simulink model "ZSM_TeslaModelS_statKreisfahrt"  (R2020b)
settings: Solver=FixedStepDiscrete  StartTime=0.0  StopTime=simtime  FixedStep=stepsize  RelTol=1e-3
undefined symbols (not defined in the file): activate_stop, activate_stop_vmax, ay_stop, ayObs, ayStiff, Bat_param, deltav_ist, DiscIntNeverNeededParam, EG_wunsch, magnitude, mu_road_LF, mu_road_LR, mu_road_RF, mu_road_RR, par_ASR, par_MDT, par_TIR, par_VEH, select_delta_h, select_M_wheel, stepsize, t, temp_betriebsstrategie, temperature_LTrange, track_left, track_right
libraries: Library_ASK x36, simulink x16, pid_lib x2, dspstat3 x2, Library_Betriebsstrategie x2, vehicle_model x2, pacejka_trans x1
(part 1 of 7)
settings Model: SimulationMode=accelerator  ExtModeTrigDuration=100  TunableVars=activate_stop,ay_stop,par_TIR,par_VEH,select_M_wheel_final,select_M_wheel_initial,select_M_wheel_time,select_delta_h_final,select_delta_h_initial,select_delta_h_time,v0  TunableVarsStorageClass=Auto,Auto,Auto,Auto,Auto,Auto,Auto,Auto,Auto,Auto,Auto  TunableVarsTypeQualifier=,,,,,,,,,,  Creator=schultze  LastModifiedBy=ga69qig
settings DataIOCC: ExternalInput=input_data  LoadExternalInput=on  SaveFormat=StructureWithTime  SaveOutput=off  DSMLogging=off  SaveTime=off  ReturnWorkspaceOutputs=off  StateSaveName=tmp_raccel_xout  SignalLoggingName=tmp_raccel_logsout
settings OptimizationCC: DefaultParameterBehavior=Inlined  ExpressionDepthLimit=2147483647  EfficientMapNaN2IntZero=off  LifeSpan=inf  SimCompilerOptimization=on
settings DebuggingCC: SignalInfNanChecking=warning  ReadBeforeWriteMsg=DisableAll  WriteAfterWriteMsg=DisableAll  WriteAfterReadMsg=DisableAll  AlgebraicLoopMsg=none  ArtificialAlgebraicLoopMsg=none  UnderspecifiedInitializationDetection=Classic  SolverPrmCheckMsg=warning  MultiTaskDSMMsg=warning  MultiTaskCondExecSysMsg=none  FcnCallInpInsideContextMsg=warning  UnconnectedInputMsg=none  UnconnectedOutputMsg=none  UnconnectedLineMsg=none  AllowSymbolicDim=off  StateNameClashWarn=warning  NonBusSignalsTreatedAsBus=warning  SFUnexpectedBacktrackingDiag=warning  SFNoUnconditionalDefaultTransitionDiag=warning  SFExecutionAtInitializationDiag=none  ArithmeticOperatorsInVariantConditions=warning
settings HardwareCC: ProdBitPerPointer=32  ProdBitPerSizeT=32  ProdBitPerPtrDiffT=32  ProdLargestAtomicFloat=None  ProdIntDivRoundTo=Undefined  ProdEndianess=Unspecified  ProdWordSize=32  ProdHWDeviceType=Generic->Unspecified (assume 32-bit Generic)  TargetBitPerPointer=64  TargetBitPerSizeT=64  TargetBitPerPtrDiffT=64  TargetLongLongMode=on  TargetIntDivRoundTo=Zero  TargetEndianess=LittleEndian  TargetWordSize=64  TargetHWDeviceType=MATLAB Host  ProdEqTarget=off
settings ModelReferenceCC: ModelReferenceMinAlgLoopOccurrences=on  PropagateSignalLabelsOutOfModel=off
settings SFSimCC: SFSimEcho=off  SimUseLocalCustomCode=off  CustomCodeUndefinedFunction=UseInterfaceOnly
settings RTWCC: SystemTargetFile=raccel.tlc  TemplateMakefile=raccel_default_tmf  RTWVerbose=off  RTWUseLocalCustomCode=off  RTWUseSimCustomCode=on
settings CodeAppCC: GenerateComments=off  MaxIdLength=128  MangleLength=10  SimulinkBlockComments=off
settings RaccelTargetCC: ENABLE_SLEXEC_SSBRIDGE=0  RTWCAPIParams=on  RTWCAPIRootIO=off
settings ConfigComp: CovMetricSettings=dw  CovSaveCumulativeToWorkspaceVar=on  CovSaveSingleToWorkspaceVar=on  CovExternalEMLEnable=off
settings SimscapeCC: SimscapeNormalizeSystem=off
settings ConfigurationSet: Description=SimMechanics 2G

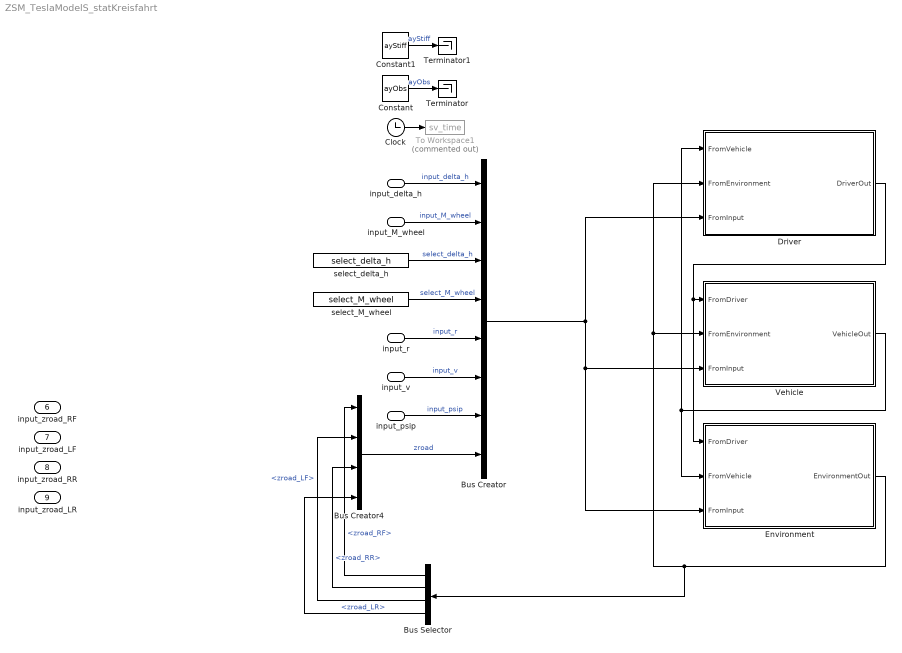
== system ZSM_TeslaModelS_statKreisfahrt ==
  input_r : Inport
  input_v : Inport  Port=2
  input_psip : Inport  Port=3
  input_delta_h : Inport  Port=4
  input_M_wheel : Inport  Port=5
  input_zroad_RF : Inport  Port=6
  input_zroad_LF : Inport  Port=7
  input_zroad_RR : Inport  Port=8
  input_zroad_LR : Inport  Port=9
  Bus Creator : BusCreator  Inputs=8
  Bus Creator4 : BusCreator  Inputs=4
  Bus Selector : BusSelector  OutputSignals=zroad_RF,zroad_RR,zroad_LF,zroad_LR
  Clock : Clock
  Constant : Constant  Value=ayObs  SampleTime=10
  Constant1 : Constant  Value=ayStiff  SampleTime=10
  Driver : Subsystem
  Environment : Subsystem
  Terminator : Terminator
  Terminator1 : Terminator
  To Workspace1 : ToWorkspace  Commented=on  VariableName=sv_time  SampleTime=-1
      settings: Decimation=savedec  Save2DSignal=2-D array (concatenate along first dimension)
  Vehicle : Subsystem
  select_M_wheel : Constant  Value=select_M_wheel
  select_delta_h : Constant  Value=select_delta_h
  wires:
  Clock/1 -> To Workspace1/1
  Bus Creator4/1 -> Bus Creator/8  "zroad"
  input_psip/1 -> Bus Creator/7  "input_psip"
  input_v/1 -> Bus Creator/6  "input_v"
  input_r/1 -> Bus Creator/5  "input_r"
  select_M_wheel/1 -> Bus Creator/4  "select_M_wheel"
  select_delta_h/1 -> Bus Creator/3  "select_delta_h"
  input_M_wheel/1 -> Bus Creator/2  "input_M_wheel"
  input_delta_h/1 -> Bus Creator/1  "input_delta_h"
  Bus Creator/1 -> Driver/3(FromInput), Environment/3(FromInput), Vehicle/3(FromInput)
  Driver/1(DriverOut) -> Environment/1(FromDriver), Vehicle/1(FromDriver)
  Vehicle/1(VehicleOut) -> Driver/1(FromVehicle), Environment/2(FromVehicle)
  Environment/1(EnvironmentOut) -> Bus Selector/1, Driver/2(FromEnvironment), Vehicle/2(FromEnvironment)
  Bus Selector/1 -> Bus Creator4/1  "<zroad_RF>"
  Bus Selector/2 -> Bus Creator4/3  "<zroad_RR>"
  Bus Selector/3 -> Bus Creator4/2  "<zroad_LF>"
  Bus Selector/4 -> Bus Creator4/4  "<zroad_LR>"
  Constant/1 -> Terminator/1  "ayObs"
  Constant1/1 -> Terminator1/1  "ayStiff"

== system ZSM_TeslaModelS_statKreisfahrt/Driver ==
  FromVehicle : Inport
  FromEnvironment : Inport  Port=2
  FromInput : Inport  Port=3
  Bus Creator : BusCreator  Inputs=2
  Bus Selector1 : BusSelector  OutputSignals=input_psip,input_r,input_delta_h,select_delta_h
  Bus Selector2 : BusSelector  OutputSignals=x.x0,y.y0,x.vx,y.vy,y.ay,psi.psi,psi.psip
  Bus Selector4 : BusSelector  OutputSignals=x.vx,x.ax,r_stat
  Bus Selector5 : BusSelector  OutputSignals=input_v,input_M_wheel,select_M_wheel
  On : Subsystem
  Splines : Subsystem
  To Workspace1 : ToWorkspace  Commented=on  VariableName=sv_FAH_delta_h1  SampleTime=-1
      settings: Decimation=savedec  Save2DSignal=2-D array (concatenate along first dimension)
  To Workspace3 : ToWorkspace  Commented=on  VariableName=sv_M_wheel  SampleTime=-1
      settings: Decimation=savedec  Save2DSignal=2-D array (concatenate along first dimension)
  driver lateral : Subsystem
  driver longitudinal : Subsystem
  DriverOut : Outport  VectorParamsAs1DForOutWhenUnconnected=off
  wires:
  Bus Creator/1 -> DriverOut/1
  FromInput/1 -> Bus Selector5/1, Bus Selector1/1
  Bus Selector2/3 -> driver lateral/3(vx)  "<vx>"
  Bus Selector2/4 -> driver lateral/4("vy ")  "<vy>"
  Bus Selector2/5 -> driver lateral/5(ay)  "<ay>"
  Bus Selector2/7 -> driver lateral/7(psip)  "<psip>"
  Bus Selector1/1 -> driver lateral/8(input_psip)  "<input_psip>"
  Bus Selector1/2 -> driver lateral/9(r soll)  "<input_r>"
  Bus Selector1/3 -> driver lateral/10(input _delta_h)  "<input_delta_h>"
  Bus Selector1/4 -> driver lateral/11(select_driver_lat)  "<select_delta_h>"
  driver longitudinal/1(M_wheel) -> Bus Creator/2, To Workspace3/1  "M_wheel"
  Bus Selector4/1 -> driver longitudinal/2(v ist)  "<vx>"
  Bus Selector5/1 -> driver longitudinal/5(v soll)  "<input_v>"
  Bus Selector5/2 -> driver longitudinal/6(input_M_wheel)  "<input_M_wheel>"
  Bus Selector5/3 -> driver longitudinal/7(select_driver_long)  "<select_M_wheel>"
  Bus Selector4/2 -> driver longitudinal/3(ax)  "<ax>"
  Bus Selector4/3 -> driver longitudinal/4(r_stat)  "<r_stat>"
  driver lateral/1(delta_h) -> Bus Creator/1, To Workspace1/1  "delta_h"
  Bus Selector2/6 -> driver lateral/6(psi)  "<psi>"
  Bus Selector2/1 -> driver lateral/1(x0)  "<x0>"
  Bus Selector2/2 -> driver lateral/2(y0)  "<y0>"
  Splines/1(Splines) -> driver longitudinal/1(Spline), driver lateral/12("spline ")
  On/1(On) -> Splines/Enable
  FromVehicle/1 -> Splines/1(Vehicle), Bus Selector4/1, Bus Selector2/1

== system ZSM_TeslaModelS_statKreisfahrt/Environment ==
  FromDriver : Inport
  FromVehicle : Inport  Port=2
  FromInput : Inport  Port=3
  Bus Creator : BusCreator  Inputs=8
  Bus Creator1 : BusCreator  Inputs=7
  Bus Creator2 : BusCreator  Inputs=4
  Bus Creator3 : BusCreator  Inputs=3
  Bus Selector : BusSelector  OutputSignals=x.vx,y.vy
  Constant{1,4..7,9..11,13..15} (11 alike) : Constant  Value=0
  Constant19 : Constant  Value=mu_road_RR
  Constant20 : Constant  Value=mu_road_LR
  Constant21 : Constant  Value=mu_road_RF
  Constant24 : Constant  Value=mu_road_LF
  Subsystem : Subsystem
  EnvironmentOut : Outport  VectorParamsAs1DForOutWhenUnconnected=off
  wires:
  Constant4/1 -> Bus Creator1/1  "init_x0"
  Constant5/1 -> Bus Creator1/2  "init_y0"
  Constant6/1 -> Bus Creator1/3  "init_psi"
  Constant7/1 -> Bus Creator1/4  "zroad_RF0"
  Constant9/1 -> Bus Creator1/5  "zroad_LF0"
  Constant10/1 -> Bus Creator1/6  "zroad_RR0"
  Constant11/1 -> Bus Creator1/7  "zroad_LR0"
  Constant21/1 -> Bus Creator2/1  "mu_road_RF"
  Constant24/1 -> Bus Creator2/2  "mu_road_LF"
  Constant19/1 -> Bus Creator2/3  "mu_road_RR"
  Constant20/1 -> Bus Creator2/4  "mu_road_LR"
  Bus Creator/1 -> EnvironmentOut/1
  Constant13/1 -> Bus Creator3/1  "vx"
  Constant14/1 -> Bus Creator3/2  "vy"
  Constant15/1 -> Bus Creator3/3  "vz"
  Bus Creator3/1 -> Bus Creator/1  "ENV_v_Wind"
  Bus Creator1/1 -> Bus Creator/3  "init_pos"
  Constant1/1 -> Bus Creator/2  "reset"
  Bus Creator2/1 -> Bus Creator/4  "ENV_road_mu"
  FromVehicle/1 -> Bus Selector/1
  Bus Selector/1 -> Subsystem/1(vx)  "<vx>"
  Bus Selector/2 -> Subsystem/2(vy)  "<vy>"
  Subsystem/1(zroad_RF) -> Bus Creator/5
  Subsystem/2(zroad_LF) -> Bus Creator/6
  Subsystem/3(zroad_RR) -> Bus Creator/7
  Subsystem/4(zroad_LR) -> Bus Creator/8

== system ZSM_TeslaModelS_statKreisfahrt/Vehicle ==
  FromDriver : Inport
  FromEnvironment : Inport  Port=2
  FromInput : Inport  Port=3
  Antriebsstrang und Radmomentenverteilung : Subsystem
  Betriebsstrategie : Subsystem
  Fahrzeugmodell : Subsystem
  VehicleOut : Outport  VectorParamsAs1DForOutWhenUnconnected=off
  wires:
  Fahrzeugmodell/1(FahrzeugmodellOut) -> VehicleOut/1, Antriebsstrang und Radmomentenverteilung/2(Ergebnisse aus dem Fahrzeugmodell), Betriebsstrategie/2(FromFahrzeugmodell)
  FromDriver/1 -> Betriebsstrategie/1(FromDriver), Fahrzeugmodell/1(FromDriver)
  FromEnvironment/1 -> Betriebsstrategie/3(FromEnvironment), Fahrzeugmodell/2(FromEnvironment)
  FromInput/1 -> Fahrzeugmodell/3(FromInput)
  Betriebsstrategie/1(BetriebsstrategieOut) -> Antriebsstrang und Radmomentenverteilung/1(Ergebnisse der Betriebsstrategie), Fahrzeugmodell/4(FromBetriebsstrategie)
  Antriebsstrang und Radmomentenverteilung/1(M_antr) -> Fahrzeugmodell/5(FromAntriebsstrang)

== system ZSM_TeslaModelS_statKreisfahrt/Driver/On ==
  Constant : Constant  Value=select_delta_h
  Constant1 : Constant  Value=4
  Relational Operator : RelationalOperator  Operator===  OutDataTypeStr=boolean  RndMeth=Simplest
  On : Outport  VectorParamsAs1DForOutWhenUnconnected=off
  wires:
  Constant/1 -> Relational Operator/1
  Constant1/1 -> Relational Operator/2
  Relational Operator/1 -> On/1

== system ZSM_TeslaModelS_statKreisfahrt/Driver/Splines ==
  Vehicle : Inport
  Enable : EnablePort
  Bus Creator : BusCreator  Inputs=8
  Bus Selector3 : BusSelector  OutputSignals=psi.psi,x.x0,y.y0
  Clock : Clock
  Constant10 : Constant  Value=t.p0
  Constant2 : Constant  Value=t.a1
  Constant3 : Constant  Value=t.a0
  Constant4 : Constant  Value=t.v2
  Constant5 : Constant  Value=t.v1
  Constant6 : Constant  Value=t.v0
  Constant7 : Constant  Value=t.p3
  Constant8 : Constant  Value=t.p2
  Constant9 : Constant  Value=t.p1
  Kennwerte : MATLAB Function  TreatAsAtomicUnit=on
  Memory : Memory
  Mux : Mux  Inputs=2
  Mux1 : Mux  Inputs=3
  Mux2 : Mux  Inputs=2
  To Workspace2 : ToWorkspace  Commented=on  VariableName=sv_SPL_pos  SampleTime=-1
      settings: Decimation=savedec  Save2DSignal=2-D array (concatenate along first dimension)
  To Workspace4 : ToWorkspace  Commented=on  VariableName=sv_SPL_delta_p  SampleTime=-1
      settings: Decimation=savedec  Save2DSignal=2-D array (concatenate along first dimension)
  Splines : Outport  VectorParamsAs1DForOutWhenUnconnected=off
  wires:
  Bus Selector3/2 -> Mux/1  "<x0>"
  Constant6/1 -> Kennwerte/7(v0)
  Constant7/1 -> Kennwerte/8(p3)
  Bus Selector3/1 -> Kennwerte/12(psi_real)  "<psi>"
  Constant9/1 -> Kennwerte/10(p1)
  Mux1/1 -> To Workspace2/1
  Kennwerte/3(spl_v_glob) -> Bus Creator/3, Mux1/2
  Clock/1 -> Kennwerte/2(time)
  Mux/1 -> Kennwerte/13(p_ist)
  Constant3/1 -> Kennwerte/4(a0)
  Vehicle/1 -> Bus Selector3/1
  Kennwerte/2(spl_a_glob) -> Bus Creator/2, Mux1/1
  Constant2/1 -> Kennwerte/3(a1)
  Kennwerte/4(spl_p_glob) -> Bus Creator/4, Mux1/3
  Bus Creator/1 -> Splines/1
  Bus Selector3/3 -> Mux/2  "<y0>"
  Mux2/1 -> To Workspace4/1
  Constant8/1 -> Kennwerte/9(p2)
  Constant5/1 -> Kennwerte/6(v1)
  Constant4/1 -> Kennwerte/5(v2)
  Constant10/1 -> Kennwerte/11(p0)
  Kennwerte/1(psi_spline) -> Bus Creator/1, Memory/1
  Memory/1 -> Kennwerte/1(psi_old)
  Kennwerte/5(spl_a_veh) -> Bus Creator/5
  Kennwerte/6(spl_v_veh) -> Bus Creator/6
  Kennwerte/7(p_err_long) -> Bus Creator/7, Mux2/1
  Kennwerte/8(p_err_lat) -> Bus Creator/8, Mux2/2

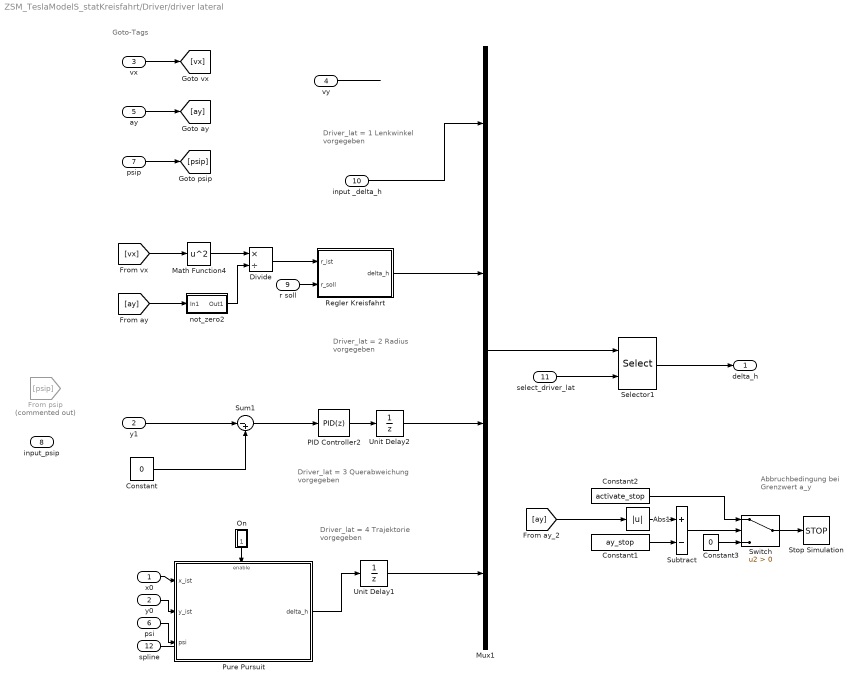
== system ZSM_TeslaModelS_statKreisfahrt/Driver/driver lateral ==
  note: Driver_lat = 1
      | Lenkwinkel vorgegeben
  note: Goto-Tags
  note: Abbruchbedingung
      | bei Grenzwert a_y
  note: Driver_lat = 3
      | Querabweichung vorgegeben
  note: Driver_lat = 2
      | Radius vorgegeben
  note: Driver_lat = 4
      | Trajektorie vorgegeben
  x0 : Inport
  y0 : Inport  Port=2
  vx : Inport  Port=3
  "vy " : Inport  Port=4
  ay : Inport  Port=5
  psi : Inport  Port=6
  psip : Inport  Port=7
  input_psip : Inport  Port=8
  r soll : Inport  Port=9
  input _delta_h : Inport  Port=10
  select_driver_lat : Inport  Port=11
  "spline " : Inport  Port=12
  Abs1 : Abs
  Constant : Constant  Value=0
  Constant1 : Constant  Value=ay_stop
  Constant2 : Constant  Value=activate_stop
  Constant3 : Constant  Value=0
  Divide : Product  Inputs=*/
  From psip : From  Commented=on  GotoTag=psip
  Math Function4 : Math  Operator=square  SignedPower=on  SaturateOnIntegerOverflow=on
  Mux1 : Mux
  On : Subsystem
  PID Controller2 : pid_lib/PID Controller  Controller=PID  Form=Parallel  TimeDomain=Discrete-time  UseExternalTs=off  SampleTime=stepsize  IntegratorMethod=Forward Euler  FilterMethod=Forward Euler  ControllerParametersSource=internal  P=10  I=10  D=8  UseFilter=on  N=1000  TunerSelectOption=Transfer Function Based (PID Tuner App)  InitialConditionSource=internal  InitialConditionForIntegrator=0  InitialConditionForFilter=0  DifferentiatorICPrevScaledInput=0  ExternalReset=none  TrackingMode=off  Kt=1  LimitOutput=off  SatLimitsSource=internal  UpperSaturationLimit=8  LowerSaturationLimit=-8  LinearizeAsGain=off  AntiWindupMode=back-calculation  Kb=1  POutMin=[]  POutMax=[]  IOutMin=[]  IOutMax=[]  DOutMin=[]  DOutMax=[]  NOutMin=[]  NOutMax=[]  SumOutMin=[]  SumOutMax=[]  SaturationOutMin=[]  SaturationOutMax=[]  PParamMin=[]  PParamMax=[]  IParamMin=[]  IParamMax=[]  DParamMin=[]  DParamMax=[]  NParamMin=[]  NParamMax=[]  KbParamMin=[]  KbParamMax=[]  KtParamMin=[]  KtParamMax=[]  KbOutMin=[]  KbOutMax=[]  KtOutMin=[]  KtOutMax=[]  IntegratorOutMin=[]  IntegratorOutMax=[]  FilterOutMin=[]  FilterOutMax=[]  SumI1OutMin=[]  SumI1OutMax=[]  SumI2OutMin=[]  SumI2OutMax=[]  SumI3OutMin=[]  SumI3OutMax=[]  SumI4OutMin=[]  SumI4OutMax=[]  SumDOutMin=[]  SumDOutMax=[]  DifferentiatorOutMin=[]  DifferentiatorOutMax=[]  FilterDiffOutCoefMin=[]  FilterDiffOutCoefMax=[]  ReciprocalOutMin=[]  ReciprocalOutMax=[]  SumDenOutMin=[]  SumDenOutMax=[]  SumNumOutMin=[]  SumNumOutMax=[]  DivideOutMin=[]  DivideOutMax=[]  UdiffTsProdOutMin=[]  UdiffTsProdOutMax=[]  NTsProdOutMin=[]  NTsProdOutMax=[]  UintegralTsProdOutMin=[]  UintegralTsProdOutMax=[]  UngainTsProdOutMin=[]  UngainTsProdOutMax=[]  IntegratorContinuousStateAttributes=''  IntegratorStateMustResolveToSignalObject=off  IntegratorRTWStateStorageClass=Auto  FilterContinuousStateAttributes=''  FilterStateMustResolveToSignalObject=off  FilterRTWStateStorageClass=Auto  ParallelPVariant=InternalParameters  IdealPVariant=Disabled  IVariant=InternalParameters  DVariant=InternalParameters  IntegratorVariant=Discrete  SatVariant=Disabled  AWVariant=Passthrough  PCopyVariant=Disabled  TRVariant=Disabled  FdbkBlocksVariant=Forward  IdealPFdbkVariant=Disabled  SatFdbkVariant=Disabled  DerivativeFilterVariant=ForwardEulerFilter  NVariant=InternalParameters  NCopyVariant=Disabled  FilterICVariant=InternalICsFilter  IntegratorICVariant=InternalICs  ExternalResetVariant=Disabled  TRSumVariant=Passthrough  SumFdbkVariant=Disabled  SumVariant=Sum_PID  TsampFilterVariant=InternalTs  TsampNgainVariant=Passthrough  TsampIntegralVariant=Passthrough  ExternalSaturationOutDataTypeStr=Inherit: Same as second input
  Pure Pursuit : Subsystem
  Regler Kreisfahrt : Subsystem
  Selector1 : Selector  InputPortWidth=4  IndexOptions=Index vector (port)  Indices=[1 3]  OutputSizes=1
  Stop Simulation : Stop
  Subtract : Sum  Inputs=+-
  Sum1 : Sum  Inputs=|-+
  Switch : Switch  Criteria=u2 > Threshold
  Unit Delay1 : UnitDelay  SampleTime=-1  HasFrameUpgradeWarning=on
  Unit Delay2 : UnitDelay  SampleTime=stepsize  HasFrameUpgradeWarning=on
  not_zero2 : Subsystem
  y1 : InportShadow  Port=2
  delta_h : Outport  VectorParamsAs1DForOutWhenUnconnected=off
  wires:
  Switch/1 -> Stop Simulation/1
  Constant1/1 -> Subtract/2
  Abs1/1 -> Subtract/1
  Subtract/1 -> Switch/2
  Constant3/1 -> Switch/3
  Constant2/1 -> Switch/1
  [vx] -> Math Function4/1
  Math Function4/1 -> Divide/1
  not_zero2/1(Out1) -> Divide/2
  Mux1/1 -> Selector1/1
  select_driver_lat/1 -> Selector1/2
  Unit Delay2/1 -> Mux1/3
  vx/1 -> [vx]
  ay/1 -> [ay]
  [ay] -> not_zero2/1(In1)
  [ay] -> Abs1/1
  psip/1 -> [psip]
  "vy "/1 -> ?
  input _delta_h/1 -> Mux1/1
  Regler Kreisfahrt/1(delta_h) -> Mux1/2
  Selector1/1 -> delta_h/1
  Divide/1 -> Regler Kreisfahrt/1(r_ist)
  r soll/1 -> Regler Kreisfahrt/2(r_soll)
  Pure Pursuit/1(delta_h) -> Unit Delay1/1
  On/1(On) -> Pure Pursuit/Enable
  "spline "/1 -> ?
  y0/1 -> Pure Pursuit/2(y_ist)
  Unit Delay1/1 -> Mux1/4
  x0/1 -> Pure Pursuit/1(x_ist)
  psi/1 -> Pure Pursuit/3(psi)
  y1/1 -> Sum1/1
  Constant/1 -> Sum1/2
  PID Controller2/1 -> Unit Delay2/1
  Sum1/1 -> PID Controller2/1

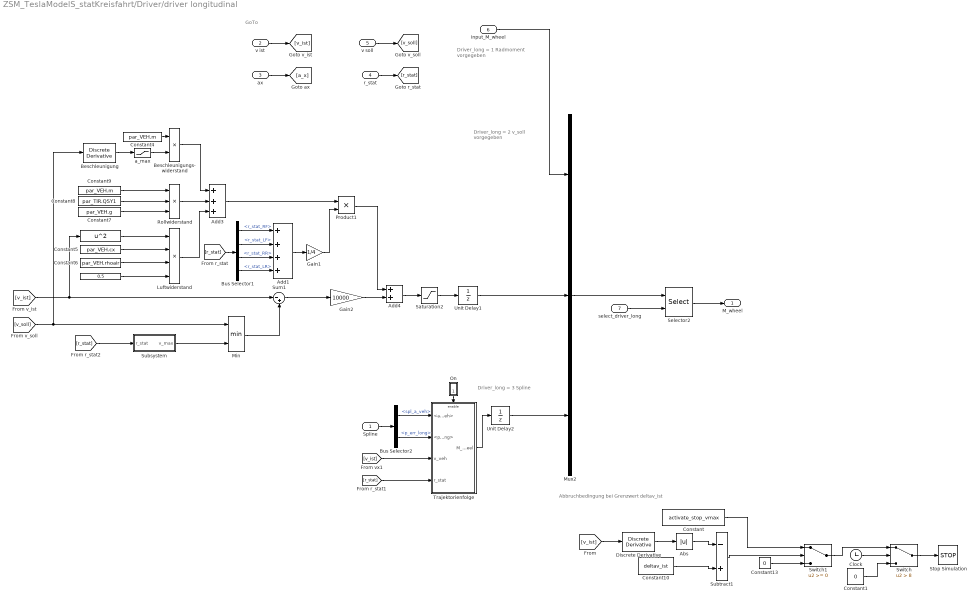
== system ZSM_TeslaModelS_statKreisfahrt/Driver/driver longitudinal ==
  note: Abbruchbedingung bei Grenzwert deltav_ist
  note: Driver_long = 3
      | Spline
  note: GoTo
  note: Driver_long = 1
      | Radmoment vorgegeben
  note: Driver_long = 2
      | v_soll vorgegeben
  Spline : Inport
  v ist : Inport  Port=2
  ax : Inport  Port=3
  r_stat : Inport  Port=4
  v soll : Inport  Port=5
  input_M_wheel : Inport  Port=6
  select_driver_long : Inport  Port=7
  " " : Constant  Value=0.5
  "  " : Math  Operator=square  SignedPower=on  SaturateOnIntegerOverflow=on
  Abs : Abs
  Add1 : Sum  Inputs=++++
  Add3 : Sum  Inputs=+++
  Add4 : Sum
  Beschleunigung : simulink/Discrete/Discrete Derivative  gainval=1.0  ICPrevScaledInput=0.0  OutMin=[]  OutMax=[]  OutDataType=fixdt(1, 16)  OutScaling=2^-10  DoSatur=off
  Beschleunigungs- widerstand : Product
  Bus Selector1 : BusSelector  OutputSignals=r_stat_RF,r_stat_LF,r_stat_RR,r_stat_LR
  Bus Selector2 : BusSelector  OutputSignals=spl_a_veh,p_err_long
  Clock : Clock
  Constant : Constant  Value=activate_stop_vmax
  Constant1 : Constant  Value=0
  Constant10 : Constant  Value=deltav_ist
  Constant13 : Constant  Value=0
  Constant4 : Constant  Value=par_VEH.m
  Constant5 : Constant  Value=par_VEH.cx
  Constant6 : Constant  Value=par_VEH.rhoair
  Constant7 : Constant  Value=par_VEH.g
  Constant8 : Constant  Value=par_TIR.QSY1
  Constant9 : Constant  Value=par_VEH.m
  Discrete Derivative : simulink/Discrete/Discrete Derivative  gainval=stepsize  ICPrevScaledInput=0  OutMin=[]  OutMax=[]  OutDataTypeStr=double  OutputDataTypeScalingMode=double  OutDataType=fixdt(1, 16)  OutScaling=2^-10  DoSatur=off
  Gain1 : Gain  Gain=1/4
  Gain2 : Gain  Gain=10000
  Luftwiderstand : Product  Inputs=4
  Min : MinMax  Inputs=2
  Mux2 : Mux  Inputs=3
  On : Subsystem
  Product1 : Product
  Rollwiderstand : Product  Inputs=3
  Saturation2 : Saturate  UpperLimit=15000  LowerLimit=-15000
  Selector2 : Selector  InputPortWidth=3  IndexOptions=Index vector (port)  Indices=[1 3]  OutputSizes=1
  Stop Simulation : Stop
  Subsystem : Subsystem
  Subtract1 : Sum  Inputs=-+
  Sum1 : Sum  Inputs=|-+
  Switch : Switch  Criteria=u2 > Threshold  Threshold=8
  Switch1 : Switch
  Trajektorienfolge : Subsystem
  Unit Delay1 : UnitDelay  SampleTime=-1  HasFrameUpgradeWarning=on
  Unit Delay2 : UnitDelay  SampleTime=stepsize  HasFrameUpgradeWarning=on
  a_max : Saturate  UpperLimit=10  LowerLimit=-10
  M_wheel : Outport  VectorParamsAs1DForOutWhenUnconnected=off
  wires:
  Selector2/1 -> M_wheel/1
  select_driver_long/1 -> Selector2/2
  input_M_wheel/1 -> Mux2/1
  Mux2/1 -> Selector2/1
  v soll/1 -> [v_soll]
  v ist/1 -> [v_ist]
  ax/1 -> [a_x]
  Sum1/1 -> Gain2/1
  [v_ist] -> "  "/1, Sum1/1
  Beschleunigungs- widerstand/1 -> Add3/1
  Rollwiderstand/1 -> Add3/2
  Constant4/1 -> Beschleunigungs- widerstand/1
  Constant8/1 -> Rollwiderstand/2
  Constant7/1 -> Rollwiderstand/3
  Luftwiderstand/1 -> Add3/3
  Constant5/1 -> Luftwiderstand/2
  Constant6/1 -> Luftwiderstand/3
  " "/1 -> Luftwiderstand/4
  "  "/1 -> Luftwiderstand/1
  Gain1/1 -> Product1/2
  Add3/1 -> Product1/1
  Beschleunigung/1 -> a_max/1
  [r_stat] -> Bus Selector1/1
  Bus Selector1/1 -> Add1/1  "<r_stat_RF>"
  Bus Selector1/3 -> Add1/3  "<r_stat_RR>"
  Bus Selector1/4 -> Add1/4  "<r_stat_LR>"
  Bus Selector1/2 -> Add1/2  "<r_stat_LF>"
  Add1/1 -> Gain1/1
  Product1/1 -> Add4/1
  Add4/1 -> Saturation2/1
  a_max/1 -> Beschleunigungs- widerstand/2
  Gain2/1 -> Add4/2
  Saturation2/1 -> Unit Delay1/1
  Constant9/1 -> Rollwiderstand/1
  r_stat/1 -> [r_stat]
  Unit Delay1/1 -> Mux2/2
  [v_soll] -> Min/1, Beschleunigung/1
  [r_stat] -> Subsystem/1(r_stat)
  Constant/1 -> Switch1/1
  [v_ist] -> Discrete Derivative/1
  Discrete Derivative/1 -> Abs/1
  Abs/1 -> Subtract1/1
  Constant10/1 -> Subtract1/2
  Subtract1/1 -> Switch1/2
  Constant13/1 -> Switch1/3
  [r_stat] -> Trajektorienfolge/4(r_stat)
  Unit Delay2/1 -> Mux2/3
  Spline/1 -> Bus Selector2/1
  Bus Selector2/1 -> Trajektorienfolge/1(<a_veh>)  "<spl_a_veh>"
  Bus Selector2/2 -> Trajektorienfolge/2(<p_long>)  "<p_err_long>"
  [v_ist] -> Trajektorienfolge/3(v_veh)
  On/1(On) -> Trajektorienfolge/Enable
  Trajektorienfolge/1(M_Wheel) -> Unit Delay2/1
  Subsystem/1(v_max) -> Min/2
  Min/1 -> Sum1/2
  Switch/1 -> Stop Simulation/1
  Switch1/1 -> Switch/1
  Clock/1 -> Switch/2
  Constant1/1 -> Switch/3

== system ZSM_TeslaModelS_statKreisfahrt/Environment/Subsystem ==
  vx : Inport
  vy : Inport  Port=2
  1-D Lookup Table : Lookup_n-D  NumberOfTableDimensions=1  BreakpointsForDimension1=[0:3000]  Table=track_right  InternalRulePriority=Speed  RndMeth=Simplest  InputSameDT=on
  1-D Lookup Table1 : Lookup_n-D  NumberOfTableDimensions=1  BreakpointsForDimension1=[0:3000]  Table=track_left  InternalRulePriority=Speed  RndMeth=Simplest  InputSameDT=on
  Add : Sum
  Add1 : Sum
  Add2 : Sum  Inputs=+-
  Constant : Constant  Value=par_VEH.xSP
  Constant2 : Constant  Value=par_VEH.l
  Constant3 : Constant  Value=0
  Demux : Demux  Outputs=2
  Demux1 : Demux  Outputs=2
  Discrete-Time Integrator : DiscreteIntegrator  SampleTime=0.01  ICPrevOutput=DiscIntNeverNeededParam  ICPrevScaledInput=DiscIntNeverNeededParam
  Math Function : Math  Operator=square  SignedPower=on  SaturateOnIntegerOverflow=on
  Math Function1 : Math  Operator=square  SignedPower=on  SaturateOnIntegerOverflow=on
  Mux : Mux  Inputs=2
  Mux1 : Mux  Inputs=2
  Product : Product
  Sign : Signum
  Sqrt : Sqrt  SaturateOnIntegerOverflow=on
  Switch : Switch  Criteria=u2 > Threshold
  zroad_RF : Outport  VectorParamsAs1DForOutWhenUnconnected=off
  zroad_LF : Outport  Port=2  VectorParamsAs1DForOutWhenUnconnected=off
  zroad_RR : Outport  Port=3  VectorParamsAs1DForOutWhenUnconnected=off
  zroad_LR : Outport  Port=4  VectorParamsAs1DForOutWhenUnconnected=off
  wires:
  Sqrt/1 -> Product/1
  Math Function1/1 -> Sign/1, Add/1
  Add/1 -> Sqrt/1
  Sign/1 -> Product/2
  Product/1 -> Discrete-Time Integrator/1
  Add1/1 -> Add2/1, Mux1/1, Mux/1
  Constant2/1 -> Add2/2
  Add2/1 -> Switch/1, Switch/2
  Constant3/1 -> Switch/3
  Discrete-Time Integrator/1 -> Add1/1
  Switch/1 -> Mux1/2, Mux/2
  Mux/1 -> 1-D Lookup Table/1
  Constant/1 -> Add1/2
  Mux1/1 -> 1-D Lookup Table1/1
  Math Function/1 -> Add/2
  Demux/1 -> zroad_RF/1  "zroad_RF"
  Demux/2 -> zroad_RR/1  "zroad_RR"
  1-D Lookup Table1/1 -> Demux1/1
  vy/1 -> Math Function/1
  vx/1 -> Math Function1/1
  Demux1/2 -> zroad_LR/1  "zroad_LR"
  1-D Lookup Table/1 -> Demux/1
  Demux1/1 -> zroad_LF/1  "zroad_LF"
